simulink model "BuckFeedbackExampleCh9PIDGvg"  (Simulink 7.5)
settings: Solver=ode45  StartTime=0.0  StopTime=10.0  RelTol=1e-3
settings Model: Creator=rwe  LastModifiedBy=rwe

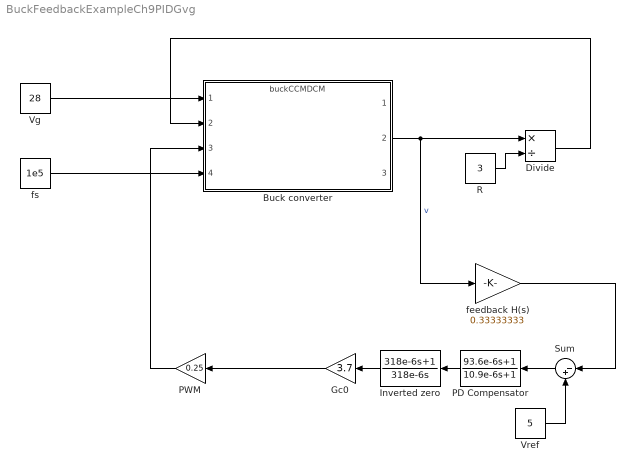
== system BuckFeedbackExampleCh9PIDGvg ==
  " Inverted zero" : TransferFcn  Numerator=[318e-6 1]  Denominator=[318e-6 0]
  Buck converter : ModelReference  ModelNameDialog=buckCCMDCM  SimulationMode=Accelerator  ModelReferenceVersion=1.26  CopyOfModelName=buckCCMDCM
  Divide : Product  Inputs=*/  OutDataType=fixdt(1, 16)  OutScaling=2^-10
  Gc0 : Gain  Gain=3.7  ParameterDataType=fixdt(1, 16)  ParameterScaling=2^0  OutDataType=fixdt(1, 16)  OutScaling=2^0
  PD Compensator : TransferFcn  Numerator=[93.6e-6 1]  Denominator=[10.9e-6 1]
  PWM : Gain  Gain=0.25  ParameterDataType=fixdt(1, 16)  ParameterScaling=2^0  OutDataType=fixdt(1, 16)  OutScaling=2^0
  R : Constant  Value=3  OutDataType=fixdt(1, 16)  OutScaling=2^0
  Sum : Sum  Inputs=|-+  OutDataType=fixdt(1, 16)  OutScaling=2^0
  Vg : Constant  Value=28  OutDataType=fixdt(1, 16)  OutScaling=2^0
  Vref : Constant  Value=5  OutDataType=fixdt(1, 16)  OutScaling=2^0
  feedback H(s) : Gain  Gain=0.33333333  ParameterDataType=fixdt(1, 16)  ParameterScaling=2^0  OutDataType=fixdt(1, 16)  OutScaling=2^0
  fs : Constant  Value=1e5  OutDataType=fixdt(1, 16)  OutScaling=2^0
  wires:
  Vg/1 -> Buck converter/1
  Buck converter/2 -> Divide/1, feedback H(s)/1  "v"
  Divide/1 -> Buck converter/2
  R/1 -> Divide/2
  fs/1 -> Buck converter/4
  feedback H(s)/1 -> Sum/1
  Vref/1 -> Sum/2
  Sum/1 -> PD Compensator/1
  PWM/1 -> Buck converter/3
  Gc0/1 -> PWM/1
  PD Compensator/1 -> " Inverted zero"/1
  " Inverted zero"/1 -> Gc0/1
